simulink model "UNIFIER_3DOFsim"  (R2023b)
settings: Solver=VariableStepAuto  StartTime=0  StopTime=t_sim  RelTol=1e-3
InitFcn:
  | UNIFIER_3DOFsim_init
values from neighbouring files (symbols this model uses):
  b = 20.11467    [UNIFIER_LOAD.m]    (also in UNIFIER_LOAD.mat; UNIFIER_LOAD_ROM.m; UNIFIER_LOAD_ROM.mat)
  c = 1.43676    [UNIFIER_LOAD.m]    (also in UNIFIER_LOAD.mat; UNIFIER_LOAD_ROM.m; UNIFIER_LOAD_ROM.mat)
  DEP_inc = -0.0872664625997    [UNIFIER_LOAD.mat]    (also in UNIFIER_ROMdyn.m = deg2rad(-5); UNIFIER_ROMdyn_script.m = deg2rad(-5); UNIFIER_ROMdyn_v2.m = deg2rad(-5); UNIFIER_ROMgen.m = 0.1)
  dp_DEP =     [UNIFIER_LOAD.mat]    (also in UNIFIER_LOAD_ROM.mat)
  dp_FUSE_FIN =     [UNIFIER_LOAD.mat]
  dp_HTU =     [UNIFIER_LOAD.mat]    (also in UNIFIER_LOAD_ROM.mat)
  dp_VTAIL =     [UNIFIER_LOAD.mat]
  dp_VTAIL_INDUCED =     [UNIFIER_LOAD.mat]
  dp_WING_root =     [UNIFIER_LOAD.mat]
  dp_WING_tip =     [UNIFIER_LOAD.mat]
  dumax = [2.09439510239 2.09439510239 2.09439510239 1.0471975512 2 4 2]    [UNIFIER_LOAD.mat]    (also in UNIFIER_LOAD_ROM.mat = [1.0471975512 1.0471975512 1.0471975512 0.174532925199 2 2 2)
  gr = 9.80665    [UNIFIER_LOAD.mat]    (also in UNIFIER_LOAD_ROM.mat)
  m = 7057    [UNIFIER_LOAD.m]    (also in UNIFIER_LOAD.mat; UNIFIER_LOAD_ROM.m; UNIFIER_LOAD_ROM.mat)
  n_prop = 12    [UNIFIER_LOAD.mat]    (also in UNIFIER_ROMdyn.m; UNIFIER_ROMdyn_script.m; UNIFIER_ROMdyn_v2.m)
  prop_d = 1.6    [UNIFIER_LOAD.mat]    (also in UNIFIER_ROMdyn.m; UNIFIER_ROMdyn_script.m; UNIFIER_ROMdyn_v2.m)
  ROMv1 = ROM    [UNIFIER_3DOFsim_init.m]    (also in UNIFIER_ROMgen_subset.m; UNIFIER_ROMgen_v2_subset.m; UNIFIER_ROMgen_v3_subset.m; UNIFIER_ROMgen_v4_subset.m)
  ROMv2 = ROM    [UNIFIER_3DOFsim_init.m]
  ROMv3 = ROM    [UNIFIER_3DOFsim_init.m]
  S = 29.98388    [UNIFIER_LOAD.m]    (also in UNIFIER_LOAD.mat; UNIFIER_LOAD_ROM.m; UNIFIER_LOAD_ROM.mat)
  U_trim = [ustar(3) ... (first row only)    [UNIFIER_3DOFsim_init.m]
  umax = inf    [UNIFIERLanding.m]    (also in UNIFIER_LOAD.mat = [0.436332312999 0.523598775598 0.523598775598 0.436332312999; UNIFIER_LOAD_ROM.mat = [0.436332312999 0.523598775598 0.349065850399 0.436332312999)
  umin = 0    [UNIFIERLanding.m]    (also in UNIFIER_LOAD.mat = [-0.436332312999 -0.523598775598 -0.523598775598 0 0 -1 -0.5; UNIFIER_LOAD_ROM.mat = [-0.436332312999 -0.523598775598 -0.0872664625997 0 0 -1 0])
  Va = sqrt(u^2+w^2)    [ROMcomp.m]    (also in UNIFIERLanding.m = sqrt(x(:,3).^2+x(:,4).^2); UNIFIERLanding_Dynamics_Internal.m = sqrt(X(:,3).^2+X(:,4).^2); UNIFIERLanding_Main.m = sqrt(solution.X(:,3).^2+solution.X(:,4).^2); UNIFIERLanding_trajopt.m = sqrt(solution.X(:,3).^2+solution.X(:,4).^2))
  vtail_nodes = [dp_VTAIL.Xs_LE;     dp_VTAIL.Ys_LE;     dp_VTAIL.Zs_LE]    [UNIFIER_LOAD.m]    (also in UNIFIER_LOAD.mat = [-16.4894695282 -2.83441376686 -2.73765826225 -16.1370849609)
  wing_nodes = [fliplr(dp_WING_tip.LE_Xs),fliplr(dp_WING_root.LE_Xs),dp_WING_root.LE_Xs,dp_WING_tip.LE_Xs;     fliplr(-dp_WING_tip.LE_Ys),fliplr(-dp_WING_root.LE_Ys),dp_WING_root.LE_Ys,dp_WING_tip.LE_Ys;     fliplr(dp_WING_tip.LE_Zs),fliplr(dp_WING_root.LE_Zs),dp_WING_root.LE_Zs,dp_WING_tip.LE_Zs]    [UNIFIER_LOAD.m]    (also in UNIFIER_LOAD.mat = [-7.70795631409 -9.67500019073 -0.98178178072 -7.66801691055)
  x0 = xstar(1)    [UNIFIERLanding.m]    (also in UNIFIER_3DOFsim_init.m; UNIFIER_dynamics.m = x; UNIFIER_trim.m = [Va_target/100; UNIFIER_trim1.m = [Va_target)
  xstar = [0;        0;        -ze_target;        zstar(1)*100;        0;        zstar(2)*100;        0;        zstar(3);        0;        0;        0;        0]    [UNIFIER_trim.m]    (also in UNIFIER_trim0_res.mat = [0 0 -500 55.1327882403 0 -0.446351795968 0 1.36591182427e-0; UNIFIER_trim1.m = [0;        0;        -ze_target;        zstar(1);        0; ; UNIFIER_trim1_res.mat = [0 0 -1219 72.7310470326 0 1.14230710452 0 0.0157060522827 0; UNIFIER_trimHFM.m = [0;        0;        -runconfig.ze;        zstar(1)*100;    )
  xyz_cg = [-8.09,0,-0.2]    [UNIFIER_LOAD.m]    (also in UNIFIER_LOAD.mat = [-8.09 0 -0.2]; UNIFIER_LOAD_ROM.m; UNIFIER_LOAD_ROM.mat = [-8.09 0 -0.2])
  xyz_cg_12 = [-8.09 0 -0.2 -8.09 0 -0.2 -8.09 0 -0.2 -8.09 0 -0.2 ... (36 elements, 3x12)]    [UNIFIER_LOAD.mat]    (also in UNIFIER_LOAD_ROM.mat)
  xyz_DEP = [ -6.9629998	-6.9210000	-6.8660002	-6.8099999	-6.7540002	-6.6999998	-6.6999998	-6.7540002	-6.8099999	-6.8660002	-6.9210000	-6.9629998 ... (first row only)    [UNIFIER_LOAD.m]    (also in UNIFIER_LOAD.mat = [-6.9629998 -10.05 -0.90899998 -6.921 -8.4499998 -0.792 -6.8; UNIFIER_LOAD_ROM.m; UNIFIER_LOAD_ROM.mat = [-6.9629998 -10.05 -0.90899998 -6.921 -8.4499998 -0.792 -6.8)
  z0 = x(1,2)    [UNIFIERLanding.m]    (also in UNIFIER_3DOFsim_init.m = xstar(3); UNIFIER_trim.m = zstar; UNIFIER_trim1.m = zstar; UNIFIER_trimHFM.m = zstar)
undefined symbols (not defined in the file or in its folder): solution
libraries: simulink_extras x17, sharedutil x5, slpidlib x4, aerolibtransform2 x4, dspindex x2, matrix_library x1, shared6dof x1, aerolibatmos2 x1, simulink x1
(part 2 of 4)

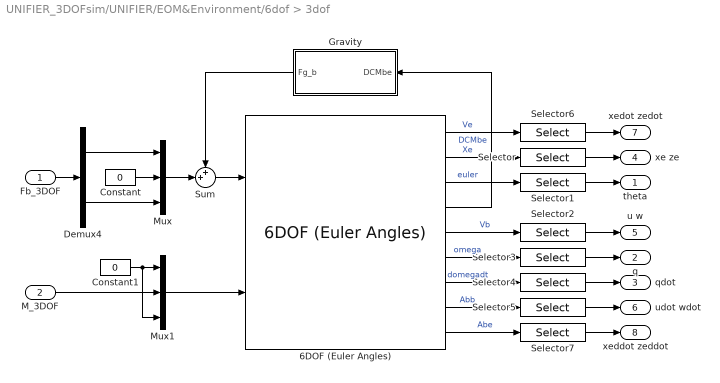
== system UNIFIER_3DOFsim/UNIFIER/EOM&Environment/6dof > 3dof ==
  Fb_3DOF : Inport
  M_3DOF : Inport  Port=2
  6DOF (Euler Angles) : shared6dof/6DOF (Euler Angles)  units=Metric (MKS)  mtype=Fixed  rep=Euler Angles  xme_0=Xe0  Vm_0=Vb0  eul_0=Euler0  pm_0=omegab0  mass_0=m  mass_e=0.5  mass_f=2.0  inertia=I  inertia_e=eye(3)  inertia_f=2*eye(3)  k_quat=1.0  vre_flag=on  abi_flag=on  aMode=0  xme_statename=''  Vm_statename=''  eul_statename=''  quat_statename=''  pm_statename=''  mass_statename=''
  Constant : Constant  Value=0
  Constant1 : Constant  Value=0
  Demux4 : Demux  Outputs=2
  Gravity : Subsystem
  Mux : Mux  Inputs=3
  Mux1 : Mux  Inputs=3
  Selector{,2,5..7} (5 alike) : Selector  InputPortWidth=3  IndexOptions=Index vector (dialog)  Indices=[1 3]  OutputSizes=1
  Selector1 : Selector  InputPortWidth=3  IndexOptions=Index vector (dialog)  Indices=[2]  OutputSizes=1
  Selector3 : Selector  InputPortWidth=3  IndexOptions=Index vector (dialog)  Indices=[2]  OutputSizes=1
  Selector4 : Selector  InputPortWidth=3  IndexOptions=Index vector (dialog)  Indices=[2]  OutputSizes=1
  Sum : Sum  Inputs=++|
  theta : Outport
  q : Outport  Port=2
  qdot : Outport  Port=3
  xe ze : Outport  Port=4
  u w : Outport  Port=5
  udot wdot : Outport  Port=6
  xedot zedot : Outport  Port=7
  xeddot zeddot : Outport  Port=8
  wires:
  Fb_3DOF/1 -> Demux4/1
  6DOF (Euler Angles)/1 -> Selector6/1  "Ve"
  Constant/1 -> Mux/2
  6DOF (Euler Angles)/9 -> Selector7/1  "Abe"
  M_3DOF/1 -> Mux1/2
  Sum/1 -> 6DOF (Euler Angles)/1
  Demux4/1 -> Mux/1
  Mux1/1 -> 6DOF (Euler Angles)/2
  Demux4/2 -> Mux/3
  Mux/1 -> Sum/2
  Gravity/1(Fg_b) -> Sum/1
  6DOF (Euler Angles)/2 -> Selector/1  "Xe"
  6DOF (Euler Angles)/4 -> Gravity/1(DCMbe)  "DCMbe"
  Constant1/1 -> Mux1/3, Mux1/1
  6DOF (Euler Angles)/3 -> Selector1/1  "euler"
  6DOF (Euler Angles)/5 -> Selector2/1  "Vb"
  6DOF (Euler Angles)/6 -> Selector3/1  "omega"
  6DOF (Euler Angles)/7 -> Selector4/1  "domegadt"
  6DOF (Euler Angles)/8 -> Selector5/1  "Abb"
  Selector/1 -> xe ze/1
  Selector1/1 -> theta/1
  Selector2/1 -> u w/1
  Selector3/1 -> q/1
  Selector4/1 -> qdot/1
  Selector5/1 -> udot wdot/1
  Selector6/1 -> xedot zedot/1
  Selector7/1 -> xeddot zeddot/1

== system UNIFIER_3DOFsim/UNIFIER/EOM&Environment/AlphaGammaVa ==
  uw : Inport
  theta : Inport  Port=2
  rho : Inport  Port=3
  Atan2 : Trigonometry  Operator=atan2
  Demux : Demux  Outputs=2
  Dot Product : DotProduct  OutDataTypeStr=Inherit: Inherit via internal rule
  Gain : Gain  Gain=1/1.225
  Product : Product
  Sqrt : Sqrt
  Sqrt1 : Sqrt
  Sum : Sum  Inputs=|+-
  alpha : Outport
  gamma : Outport  Port=2
  Va_tas : Outport  Port=3
  Va_eas : Outport  Port=4
  wires:
  uw/1 -> Dot Product/2, Dot Product/1, Demux/1
  Demux/2 -> Atan2/1
  Atan2/1 -> Sum/2, alpha/1
  theta/1 -> Sum/1
  Sum/1 -> gamma/1
  Demux/1 -> Atan2/2
  Dot Product/1 -> Sqrt/1
  Sqrt/1 -> Product/1, Va_tas/1
  Sqrt1/1 -> Product/2
  Product/1 -> Va_eas/1
  Gain/1 -> Sqrt1/1
  rho/1 -> Gain/1

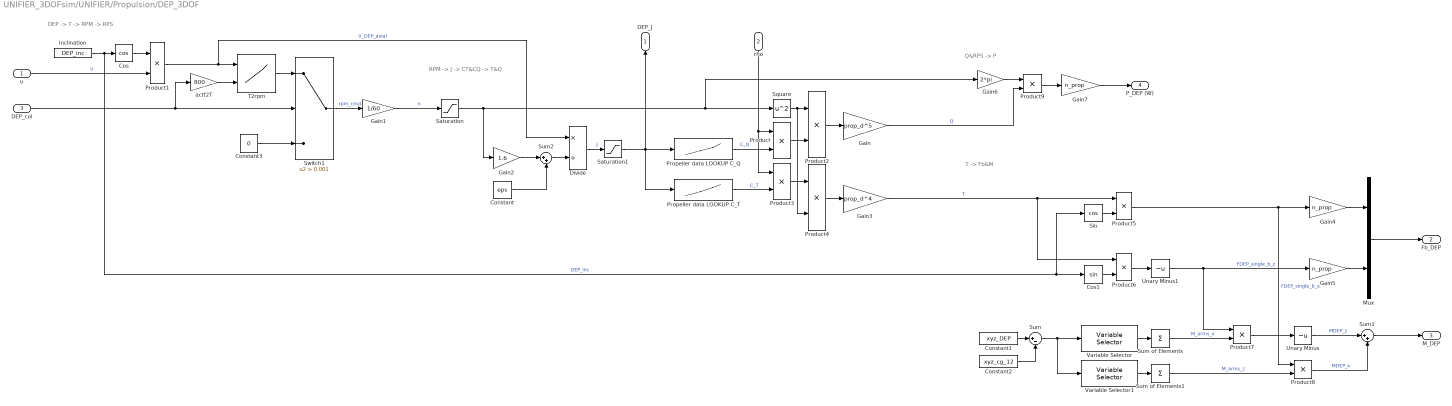
== system UNIFIER_3DOFsim/UNIFIER/Propulsion/DEP_3DOF ==
  note: Q&RPS -> P
  note: T -> Fb&M
  note: RPM -> J -> CT&CQ -> T&Q
  note: DEP -> T -> RPM -> RPS
  u : Inport
  rho : Inport  Port=2
  DEP_col : Inport  Port=3
  Constant : Constant  Value=eps
  Constant1 : Constant  Value=xyz_DEP
  Constant2 : Constant  Value=xyz_cg_12
  Constant3 : Constant  Value=0
  Cos : Trigonometry  Operator=cos
  Cos1 : Trigonometry
  Divide : Product  Inputs=*/
  Gain : Gain  Gain=prop_d^5
  Gain1 : Gain  Gain=1/60
  Gain2 : Gain  Gain=1.6
  Gain3 : Gain  Gain=prop_d^4
  Gain4 : Gain  Gain=n_prop
  Gain5 : Gain  Gain=n_prop
  Gain6 : Gain  Gain=2*pi
  Gain7 : Gain  Gain=n_prop
  Inclination : Constant  Value=DEP_inc
  Mux : Mux  Inputs=2
  Product{,1..9} (10 alike) : Product
  Propeller data LOOKUP C_Q : Lookup_n-D  NumberOfTableDimensions=1  BreakpointsForDimension1=dp_DEP.J  IndexSearchMethod=Linear search  BeginIndexSearchUsingPreviousIndexResult=on  Table=dp_DEP.C_Q  ExtrapMethod=Clip  UseLastTableValue=on  InternalRulePriority=Speed  RndMeth=Simplest
  Propeller data LOOKUP C_T : Lookup_n-D  NumberOfTableDimensions=1  BreakpointsForDimension1=dp_DEP.J  IndexSearchMethod=Linear search  BeginIndexSearchUsingPreviousIndexResult=on  Table=dp_DEP.C_T  ExtrapMethod=Clip  UseLastTableValue=on  InternalRulePriority=Speed  RndMeth=Simplest
  Saturation : Saturate  UpperLimit=inf  LowerLimit=0
  Saturation1 : Saturate  UpperLimit=2.5  LowerLimit=0.3
  Sin : Trigonometry  Operator=cos
  Square : Math  Operator=square
  Sum : Sum  Inputs=|+-
  Sum of Elements : Sum  Inputs=+
  Sum of Elements1 : Sum  Inputs=+
  Sum1 : Sum  Inputs=|++
  Sum2 : Sum  Inputs=|++
  Switch1 : Switch  Criteria=u2 > Threshold  Threshold=0.001  SaturateOnIntegerOverflow=off  InputSameDT=off
  T2rpm : Lookup_n-D  BreakpointsForDimension1=dp_DEP.rpm_lookup.V_vec  BreakpointsForDimension2=dp_DEP.rpm_lookup.T_vec  IndexSearchMethod=Linear search  BeginIndexSearchUsingPreviousIndexResult=on  Table=dp_DEP.rpm_lookup.rpm_gird  ExtrapMethod=Clip  InternalRulePriority=Speed  RndMeth=Simplest
      settings: InputPortMap=u0,u1
  Unary Minus : UnaryMinus
  Unary Minus1 : UnaryMinus
  Variable Selector : dspindex/Variable Selector  NumInputs=1  rowsOrCols=Rows  IdxMode=Fixed  Elements=[1]  ZerOneIdxMode=One-based  errmode=Clip Index  FillMode=on  FillValues=0
  Variable Selector1 : dspindex/Variable Selector  NumInputs=1  rowsOrCols=Rows  IdxMode=Fixed  Elements=[3]  ZerOneIdxMode=One-based  errmode=Clip Index  FillMode=on  FillValues=0
  actf2T : Gain  Gain=800
  DEP_J : Outport
  Fb_DEP : Outport  Port=2
  M_DEP : Outport  Port=3
  P_DEP (W) : Outport  Port=4
  wires:
  Cos/1 -> Product1/1
  Inclination/1 -> Cos1/1, Sin/1, Cos/1  "DEP_inc"
  u/1 -> Product1/2  "u"
  Constant2/1 -> Sum/2
  Constant1/1 -> Sum/1
  Constant3/1 -> Switch1/3
  T2rpm/1 -> Switch1/1
  actf2T/1 -> T2rpm/2
  Product1/1 -> Divide/1, T2rpm/1  "V_DEP_axial"
  DEP_col/1 -> actf2T/1, Switch1/2
  Switch1/1 -> Gain1/1  "rpm_cmd"
  Gain1/1 -> Saturation/1  "n"
  Product2/1 -> Gain/1
  Product4/1 -> Gain3/1
  Gain3/1 -> Product6/1, Product5/1  "T"
  Gain2/1 -> Sum2/1
  Constant/1 -> Sum2/2
  Gain/1 -> Product9/2  "Q"
  Saturation/1 -> Gain2/1, Square/1, Gain6/1
  Divide/1 -> Saturation1/1  "J"
  Saturation1/1 -> Propeller data LOOKUP C_Q/1, Propeller data LOOKUP C_T/1, DEP_J/1
  Product/1 -> Product2/2
  Propeller data LOOKUP C_T/1 -> Product3/2  "C_T"
  Propeller data LOOKUP C_Q/1 -> Product/2  "C_Q"
  Square/1 -> Product2/1, Product4/2
  Product3/1 -> Product4/1
  rho/1 -> Product/1, Product3/1
  Sum2/1 -> Divide/2
  Sum/1 -> Variable Selector1/1, Variable Selector/1
  Variable Selector/1 -> Sum of Elements/1
  Variable Selector1/1 -> Sum of Elements1/1
  Sum of Elements/1 -> Product7/2  "M_arms_x"
  Sum of Elements1/1 -> Product8/2  "M_arms_z"
  Sin/1 -> Product5/2
  Cos1/1 -> Product6/2
  Product5/1 -> Product8/1, Gain4/1  "FDEP_single_b_x"
  Product6/1 -> Unary Minus1/1
  Unary Minus1/1 -> Product7/1, Gain5/1  "FDEP_single_b_z"
  Gain4/1 -> Mux/1
  Gain5/1 -> Mux/2
  Mux/1 -> Fb_DEP/1
  Product7/1 -> Unary Minus/1
  Unary Minus/1 -> Sum1/1  "MDEP_z"
  Product8/1 -> Sum1/2  "MDEP_x"
  Sum1/1 -> M_DEP/1
  Gain6/1 -> Product9/1
  Product9/1 -> Gain7/1
  Gain7/1 -> P_DEP (W)/1

== system UNIFIER_3DOFsim/UNIFIER/Propulsion/HTU ==
  Va_eas : Inport
  HTU : Inport  Port=2
  1-D Lookup Table1 : Lookup_n-D  NumberOfTableDimensions=1  BreakpointsForDimension1=[-0.5,1.5]  IndexSearchMethod=Linear search  BeginIndexSearchUsingPreviousIndexResult=on  Table=[-5000, 15000]  ExtrapMethod=Clip  InternalRulePriority=Speed  RndMeth=Simplest
  Constant : Constant  Value=0
  Gain : Gain  Gain=1/0.92
  Gain1 : Gain  Gain=1000
  Mux : Mux  Inputs=2
  PropAndMotor : Subsystem
  Fb_HTU : Outport
  M_HTU : Outport  Port=2
  P_HTU (W) : Outport  Port=3
  wires:
  Gain/1 -> Gain1/1  "P(kW)"
  HTU/1 -> 1-D Lookup Table1/1
  1-D Lookup Table1/1 -> PropAndMotor/2(T_cmd (N))
  Va_eas/1 -> PropAndMotor/1(Vrw_mag_eas)
  PropAndMotor/1(P (kW)) -> Gain/1
  PropAndMotor/2(T (N)) -> Mux/1
  Mux/1 -> Fb_HTU/1
  Constant/1 -> M_HTU/1, Mux/2
  Gain1/1 -> P_HTU (W)/1

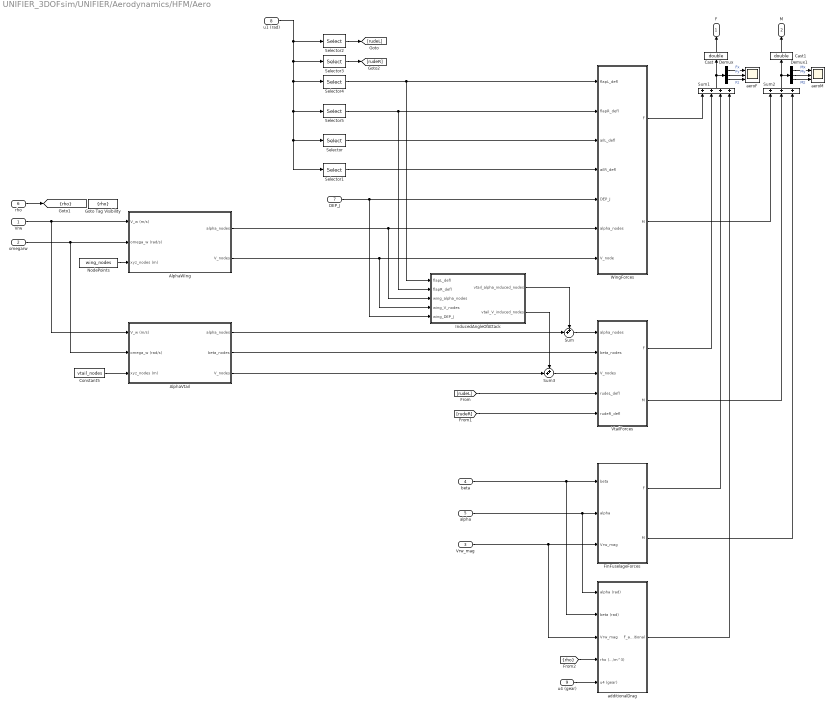
== system UNIFIER_3DOFsim/UNIFIER/Aerodynamics/HFM/Aero ==
  Vrw : Inport  OutDataTypeStr=single  Unit=m/s  PortDimensions=3  LockScale=on
  omegarw : Inport  Port=2  OutDataTypeStr=single  Unit=rad/s  PortDimensions=3  LockScale=on
  Vrw_mag : Inport  Port=3  OutDataTypeStr=single
  beta : Inport  Port=4  OutDataTypeStr=single
  alpha : Inport  Port=5  OutDataTypeStr=single
  rho : Inport  Port=6  OutDataTypeStr=single  Unit=kg/m^3  PortDimensions=1  LockScale=on
  DEP_J : Inport  Port=7  OutDataTypeStr=single  PortDimensions=12  LockScale=on
  u1 (rad) : Inport  Port=8
  u4 (gear) : Inport  Port=9
  AlphaVtail : Subsystem  TreatAsAtomicUnit=on
  AlphaWIng : Subsystem  TreatAsAtomicUnit=on
  Cast : DataTypeConversion  OutDataTypeStr=double  SaturateOnIntegerOverflow=off  RndMeth=Floor
  Cast1 : DataTypeConversion  OutDataTypeStr=double  SaturateOnIntegerOverflow=off  RndMeth=Floor
  Constant5 : Constant  Value=vtail_nodes
  Demux : Demux  Outputs=3
  Demux1 : Demux  Outputs=3
  FinFuselageForces : Subsystem
  Goto Tag Visibility : GotoTagVisibility  GotoTag=rho
  InducedAngleOfAttack : Subsystem
  NodePoints : Constant  Value=wing_nodes
  Selector : Selector  InputPortWidth=6  IndexOptions=Index vector (dialog)  Indices=1  OutputSizes=1
  Selector1 : Selector  InputPortWidth=6  IndexOptions=Index vector (dialog)  Indices=2  OutputSizes=1
  Selector2 : Selector  InputPortWidth=6  IndexOptions=Index vector (dialog)  Indices=3  OutputSizes=1
  Selector3 : Selector  InputPortWidth=6  IndexOptions=Index vector (dialog)  Indices=4  OutputSizes=1
  Selector4 : Selector  InputPortWidth=6  IndexOptions=Index vector (dialog)  Indices=5  OutputSizes=1
  Selector5 : Selector  InputPortWidth=6  IndexOptions=Index vector (dialog)  Indices=6  OutputSizes=1
  Sum : Sum  Inputs=++|
  Sum1 : Sum  Inputs=++++
  Sum2 : Sum  Inputs=+++
  Sum3 : Sum  Inputs=++|
  VtailForces : Subsystem
  WingForces : Subsystem
  additionalDrag : Subsystem
  aeroF : Scope  NumInputPorts=3
  aeroM : Scope  NumInputPorts=3
  F : Outport  Unit=N  PortDimensions=3  LockScale=on
  M : Outport  Port=2  Unit=N*m  PortDimensions=3  LockScale=on
  tag scope: rho=scoped
  wires:
  u1 (rad)/1 -> Selector2/1, Selector3/1, Selector4/1, Selector5/1, Selector/1, Selector1/1
  u4 (gear)/1 -> additionalDrag/5(u4 (gear))
  additionalDrag/1(F_additional) -> Sum1/4
  [rho] -> additionalDrag/4(rho (kg/m^3))
  alpha/1 -> FinFuselageForces/2(alpha), additionalDrag/1(alpha (rad))
  AlphaWIng/1(alpha_nodes) -> InducedAngleOfAttack/3(wing_alpha_nodes), WingForces/6(alpha_nodes)
  Demux1/3 -> aeroM/3  "Mz"
  Demux1/1 -> aeroM/1  "Mx"
  Demux1/2 -> aeroM/2  "My"
  Sum2/1 -> Demux1/1, Cast1/1
  Demux/3 -> aeroF/3  "Fz"
  Demux/2 -> aeroF/2  "Fy"
  Demux/1 -> aeroF/1  "Fx"
  Selector3/1 -> [rudeR]
  Selector2/1 -> [rudeL]
  Selector5/1 -> InducedAngleOfAttack/2(flapR_defl), WingForces/2(flapR_defl)
  Selector4/1 -> InducedAngleOfAttack/1(flapL_defl), WingForces/1(flapL_defl)
  Selector1/1 -> WingForces/4(ailR_defl)
  Selector/1 -> WingForces/3(ailL_defl)
  FinFuselageForces/2(M) -> Sum2/3
  FinFuselageForces/1(F) -> Sum1/3
  beta/1 -> FinFuselageForces/1(beta), additionalDrag/2(beta (rad))
  Vrw_mag/1 -> FinFuselageForces/3(Vrw_mag), additionalDrag/3(Vrw_mag)
  Cast1/1 -> M/1
  Cast/1 -> F/1
  AlphaVtail/1(alpha_nodes) -> Sum/2
  Sum3/1 -> VtailForces/3(V_nodes)
  InducedAngleOfAttack/2(vtail_V_induced_nodes) -> Sum3/1
  InducedAngleOfAttack/1(vtail_alpha_induced_nodes) -> Sum/1
  AlphaVtail/3(V_nodes) -> Sum3/2
  Sum1/1 -> Cast/1, Demux/1
  VtailForces/2(M) -> Sum2/2
  WingForces/2(M) -> Sum2/1
  VtailForces/1(F) -> Sum1/2
  WingForces/1(F) -> Sum1/1
  [rudeR] -> VtailForces/5(rudeR_defl)
  [rudeL] -> VtailForces/4(rudeL_defl)
  AlphaVtail/2(beta_nodes) -> VtailForces/2(beta_nodes)
  rho/1 -> [rho]
  Sum/1 -> VtailForces/1(alpha_nodes)
  DEP_J/1 -> InducedAngleOfAttack/5(wing_DEP_J), WingForces/5(DEP_J)
  AlphaWIng/2(V_nodes) -> InducedAngleOfAttack/4(wing_V_nodes), WingForces/7(V_node)
  omegarw/1 -> AlphaWIng/2(omega_w (rad/s)), AlphaVtail/2(omega_w (rad/s))
  Vrw/1 -> AlphaWIng/1(V_w (m/s)), AlphaVtail/1(V_w (m/s))
  Constant5/1 -> AlphaVtail/3(xyz_nodes (m))
  NodePoints/1 -> AlphaWIng/3(xyz_nodes (m))

== system UNIFIER_3DOFsim/UNIFIER/Aerodynamics/HFM/FillControls ==
  U_3dof : Inport
  Constant : Constant  Value=0
  Demux : Demux
  Mux : Mux  Inputs=7
  U_6dof : Outport
  wires:
  Constant/1 -> Mux/1, Mux/2, Mux/6  "ail, rud, DEP_slp"
  Mux/1 -> U_6dof/1
  U_3dof/1 -> Demux/1
  Demux/1 -> Mux/3  "elev"
  Demux/2 -> Mux/4  "flap"
  Demux/3 -> Mux/5  "DEP_col"
  Demux/4 -> Mux/7  "HTU"

== system UNIFIER_3DOFsim/UNIFIER/Aerodynamics/HFM/FillStates ==
  X_3dof : Inport
  Bus Selector : BusSelector  OutputSignals=q,theta,w,u,ze,xe
  Constant : Constant  Value=0
  Mux : Mux  Inputs=12
  X_6dof : Outport
  wires:
  X_3dof/1 -> Bus Selector/1
  Bus Selector/6 -> Mux/1  "<xe>"
  Mux/1 -> X_6dof/1
  Bus Selector/5 -> Mux/3  "<ze>"
  Bus Selector/4 -> Mux/4  "<u>"
  Bus Selector/3 -> Mux/6  "<w>"
  Bus Selector/2 -> Mux/8  "<theta>"
  Bus Selector/1 -> Mux/11  "<q>"
  Constant/1 -> Mux/12, Mux/10, Mux/9, Mux/5, Mux/2, Mux/7

== system UNIFIER_3DOFsim/UNIFIER/Aerodynamics/HFM/Ganging ==
  U_ganged : Inport
  Constant : Constant  Value=0
  Demux : Demux  Outputs=7
  For Each Subsystem : Subsystem  TreatAsAtomicUnit=on
  Mux : Mux  Inputs=2
  Mux1 : Mux  Inputs=2
  Mux2 : Mux  Inputs=2
  Mux3 : Mux
  Mux4 : Mux  Inputs=3
  Unary Minus : UnaryMinus
  V-tail mixing : Subsystem
  zeta : Constant  Value=[-1, -0.8, -0.4, -0.2, -0.1, 0, 0, 0.1, 0.2, 0.4, 0.8, 1]
  U_all : Outport
  wires:
  U_ganged/1 -> Demux/1
  Mux3/1 -> U_all/1
  Demux/1 -> Mux/1, Unary Minus/1  "ail"
  Unary Minus/1 -> Mux/2
  V-tail mixing/1(rudL) -> Mux1/1
  V-tail mixing/2(rudR) -> Mux1/2
  Demux/4 -> Mux2/2, Mux2/1  "flap"
  Demux/7 -> Mux3/3  "u3"
  Mux/1 -> Mux4/1  "ail"
  Mux1/1 -> Mux4/2  "rud"
  Mux2/1 -> Mux4/3  "flap"
  Demux/5 -> For Each Subsystem/2(DEP_col)  "DEP_col"
  Demux/6 -> For Each Subsystem/3(DEP_slope)  "DEP_slp"
  For Each Subsystem/1(Out1) -> Mux3/2  "u2"
  Mux4/1 -> Mux3/1  "u1"
  Constant/1 -> Mux3/4  "u4"
  zeta/1 -> For Each Subsystem/1(zeta)
  Demux/2 -> V-tail mixing/1(rud)  "rud"
  Demux/3 -> V-tail mixing/2(elev)  "elev"

== system UNIFIER_3DOFsim/UNIFIER/Aerodynamics/HFM/Subsystem ==
  In1 : Inport
  Mux : Mux  Inputs=12
  Out1 : Outport
  wires:
  Mux/1 -> Out1/1
  In1/1 -> Mux/3, Mux/4, Mux/5, Mux/6, Mux/7, Mux/8, Mux/9, Mux/10, Mux/11, Mux/12, Mux/2, Mux/1

== system UNIFIER_3DOFsim/UNIFIER/Aerodynamics/ROM/ROMv1 ==
  alpha : Inport
  elev : Inport  Port=2
  flap : Inport  Port=3
  J : Inport  Port=4
  n-D Lookup Table : Lookup_n-D  NumberOfTableDimensions=4  BreakpointsForDimension1=ROMv1.dFlap  BreakpointsForDimension2=ROMv1.alpha  BreakpointsForDimension3=ROMv1.J  BreakpointsForDimension4=ROMv1.dElev  Table=ROMv1.CL  InternalRulePriority=Speed  RndMeth=Simplest
      settings: InputPortMap=u0,u1,u2,u3
  n-D Lookup Table1 : Lookup_n-D  NumberOfTableDimensions=4  BreakpointsForDimension1=ROMv1.dFlap  BreakpointsForDimension2=ROMv1.alpha  BreakpointsForDimension3=ROMv1.J  BreakpointsForDimension4=ROMv1.dElev  Table=ROMv1.CD  InternalRulePriority=Speed  RndMeth=Simplest
      settings: InputPortMap=u0,u1,u2,u3
  n-D Lookup Table2 : Lookup_n-D  NumberOfTableDimensions=4  BreakpointsForDimension1=ROMv1.dFlap  BreakpointsForDimension2=ROMv1.alpha  BreakpointsForDimension3=ROMv1.J  BreakpointsForDimension4=ROMv1.dElev  Table=ROMv1.CM  InternalRulePriority=Speed  RndMeth=Simplest
      settings: InputPortMap=u0,u1,u2,u3
  CL : Outport
  CD : Outport  Port=2
  CM : Outport  Port=3
  wires:
  n-D Lookup Table/1 -> CL/1
  n-D Lookup Table1/1 -> CD/1
  n-D Lookup Table2/1 -> CM/1
  flap/1 -> n-D Lookup Table/1, n-D Lookup Table2/1, n-D Lookup Table1/1
  alpha/1 -> n-D Lookup Table/2, n-D Lookup Table2/2, n-D Lookup Table1/2
  J/1 -> n-D Lookup Table2/3, n-D Lookup Table/3, n-D Lookup Table1/3
  elev/1 -> n-D Lookup Table2/4, n-D Lookup Table1/4, n-D Lookup Table/4

== system UNIFIER_3DOFsim/UNIFIER/Aerodynamics/ROM/ROMv2 ==
  alpha : Inport
  elev : Inport  Port=2
  flap : Inport  Port=3
  n-D Lookup Table : Lookup_n-D  NumberOfTableDimensions=3  BreakpointsForDimension1=ROMv2.alpha  BreakpointsForDimension2=ROMv2.dElev  BreakpointsForDimension3=ROMv2.dFlap  Table=ROMv2.CL  InternalRulePriority=Speed  RndMeth=Simplest
      settings: InputPortMap=u0,u1,u2
  n-D Lookup Table1 : Lookup_n-D  NumberOfTableDimensions=3  BreakpointsForDimension1=ROMv2.alpha  BreakpointsForDimension2=ROMv2.dElev  BreakpointsForDimension3=ROMv2.dFlap  Table=ROMv2.CD  InternalRulePriority=Speed  RndMeth=Simplest
      settings: InputPortMap=u0,u1,u2
  n-D Lookup Table2 : Lookup_n-D  NumberOfTableDimensions=3  BreakpointsForDimension1=ROMv2.alpha  BreakpointsForDimension2=ROMv2.dElev  BreakpointsForDimension3=ROMv2.dFlap  Table=ROMv2.CM  InternalRulePriority=Speed  RndMeth=Simplest
      settings: InputPortMap=u0,u1,u2
  CL : Outport
  CD : Outport  Port=2
  CM : Outport  Port=3
  wires:
  alpha/1 -> n-D Lookup Table/1, n-D Lookup Table2/1, n-D Lookup Table1/1
  elev/1 -> n-D Lookup Table2/2, n-D Lookup Table1/2, n-D Lookup Table/2
  flap/1 -> n-D Lookup Table2/3, n-D Lookup Table1/3, n-D Lookup Table/3
  n-D Lookup Table/1 -> CL/1
  n-D Lookup Table1/1 -> CD/1
  n-D Lookup Table2/1 -> CM/1

== system UNIFIER_3DOFsim/UNIFIER/Aerodynamics/ROM/ROMv3 ==
  alpha : Inport
  elev : Inport  Port=2
  1-D Lookup Table : Lookup_n-D  NumberOfTableDimensions=1  BreakpointsForDimension1=ROMv3.alpha  Table=ROMv3.CL  InternalRulePriority=Speed  RndMeth=Simplest
  1-D Lookup Table1 : Lookup_n-D  NumberOfTableDimensions=1  BreakpointsForDimension1=ROMv3.alpha  Table=ROMv3.CD  InternalRulePriority=Speed  RndMeth=Simplest
  2-D Lookup Table : Lookup_n-D  LookupTableObject=''  BreakpointsForDimension1=ROMv3.alpha  BreakpointsForDimension2=ROMv3.dElev  BreakpointsForDimension1FirstPoint=10  BreakpointsForDimension2FirstPoint=10  BreakpointsForDimension1Spacing=12  BreakpointsForDimension2Spacing=12  IndexSearchMethod=Evenly spaced points  Table=ROMv3.CM  InterpMethod=Flat  DiagnosticForOutOfRangeInput=Error  InternalRulePriority=Speed  RndMeth=Simplest
      settings: InputPortMap=u0,u1
  CL : Outport
  CD : Outport  Port=2
  CM : Outport  Port=3
  wires:
  alpha/1 -> 1-D Lookup Table/1, 2-D Lookup Table/1, 1-D Lookup Table1/1
  elev/1 -> 2-D Lookup Table/2
  1-D Lookup Table/1 -> CL/1
  1-D Lookup Table1/1 -> CD/1
  2-D Lookup Table/1 -> CM/1

== system UNIFIER_3DOFsim/UNIFIER/Aerodynamics/ROM/calcDynamicPresure ==
  rho : Inport
  Va : Inport  Port=2
  Gain : Gain  Gain=0.5
  Product : Product
  Square : Math  Operator=square
  Q : Outport
  wires:
  Va/1 -> Square/1
  Square/1 -> Product/1
  rho/1 -> Gain/1
  Gain/1 -> Product/2
  Product/1 -> Q/1

== system UNIFIER_3DOFsim/UNIFIER/Aerodynamics/ROM/wind2body ==
  L : Inport
  D : Inport  Port=2
  alpha : Inport  Port=3
  Cos : Trigonometry  Operator=cos
  Product{,1..3} (4 alike) : Product
  Sin : Trigonometry
  Sum : Sum  Inputs=|+-
  Sum1 : Sum  Inputs=|++
  Unary Minus : UnaryMinus
  Unary Minus1 : UnaryMinus
  Fb_ae_x : Outport
  Fb_ae_z : Outport  Port=2
  wires:
  alpha/1 -> Sin/1, Cos/1
  Unary Minus/1 -> Fb_ae_x/1
  Unary Minus1/1 -> Fb_ae_z/1
  Cos/1 -> Product3/1, Product/1
  D/1 -> Product/2, Product2/2
  Sin/1 -> Product1/1, Product2/1
  L/1 -> Product3/2, Product1/2
  Product/1 -> Sum/1  "Dcos(alpha)"
  Product1/1 -> Sum/2  "Lsin(alpha)"
  Sum/1 -> Unary Minus/1
  Product2/1 -> Sum1/1  "Dsin(alpha)"
  Product3/1 -> Sum1/2  "Lcos(alpha)"
  Sum1/1 -> Unary Minus1/1

== system UNIFIER_3DOFsim/UNIFIER/EOM&Environment/6dof > 3dof/Gravity ==
  DCMbe : Inport
  Constant1 : Constant  Value=m*gr
  Constant3 : Constant  Value=0
  Product3 : Product  Multiplication=Matrix(*)
  Vector Concatenate1 : Concatenate  NumInputs=3
  Fg_b : Outport
  wires:
  DCMbe/1 -> Product3/1
  Constant1/1 -> Vector Concatenate1/3
  Constant3/1 -> Vector Concatenate1/2, Vector Concatenate1/1
  Vector Concatenate1/1 -> Product3/2
  Product3/1 -> Fg_b/1  "F"

== system UNIFIER_3DOFsim/UNIFIER/Propulsion/HTU/PropAndMotor ==
  Vrw_mag_eas : Inport
  T_cmd (N) : Inport  Port=2
  1-D Lookup Table : Lookup_n-D  NumberOfTableDimensions=1  BreakpointsForDimension1=dp_HTU.limits.V_low_lim  IndexSearchMethod=Linear search  BeginIndexSearchUsingPreviousIndexResult=on  Table=dp_HTU.limits.T_low_lim  InternalRulePriority=Speed  RndMeth=Simplest
  1-D Lookup Table1 : Lookup_n-D  NumberOfTableDimensions=1  BreakpointsForDimension1=dp_HTU.limits.V_up_lim  IndexSearchMethod=Linear search  BeginIndexSearchUsingPreviousIndexResult=on  Table=dp_HTU.limits.T_up_lim  InternalRulePriority=Speed  RndMeth=Simplest
  P lookup : Lookup_n-D  BreakpointsForDimension1=dp_HTU.V_vec  BreakpointsForDimension2=dp_HTU.T_vec  IndexSearchMethod=Linear search  BeginIndexSearchUsingPreviousIndexResult=on  Table=dp_HTU.P_grid  InternalRulePriority=Speed  RndMeth=Simplest
      settings: InputPortMap=u0,u1
  Saturation Dynamic : simulink/Discontinuities/Saturation Dynamic  OutMin=[]  OutMax=[]  OutDataTypeStr=Inherit: Same as second input  OutDataType=fixdt(1, 16)  OutScaling=2^-10  DoSatur=off
  P (kW) : Outport
  T (N) : Outport  Port=2
  wires:
  Saturation Dynamic/1 -> P lookup/2, T (N)/1
  T_cmd (N)/1 -> Saturation Dynamic/2
  1-D Lookup Table/1 -> Saturation Dynamic/3
  1-D Lookup Table1/1 -> Saturation Dynamic/1
  P lookup/1 -> P (kW)/1
  Vrw_mag_eas/1 -> P lookup/1, 1-D Lookup Table1/1, 1-D Lookup Table/1

== system UNIFIER_3DOFsim/UNIFIER/Aerodynamics/HFM/Aero/AlphaVtail ==
  V_w (m/s) : Inport
  omega_w (rad/s) : Inport  Port=2
  xyz_nodes (m) : Inport  Port=3  Partition=on  PartitionDimension=2  PartitionWidth=1  PartitionOffset=0
  3x3 Cross Product : sharedutil/3x3 Cross Product  aMode=aMode
  Asin : Trigonometry  Operator=asin
  Atan : Trigonometry  Operator=atan
  Cast : DataTypeConversion  OutDataTypeStr=single  SaturateOnIntegerOverflow=off  RndMeth=Floor
  Constant : Constant  Value=xyz_cg
  Constant1 : Constant  Value=eps  OutDataTypeStr=single
  Demux : Demux  Outputs=3
  Divide : Product  Inputs=*/
  Divide1 : Product  Inputs=*/
  For Each : ForEach  DisableCoverage=on  SpecifiedNumIters=16
  Mux : Mux  Inputs=3
  Sum : Sum  Inputs=+-
  Sum1 : Sum  Inputs=++|
  Sum2 : Sum  Inputs=|++
  Sum3 : Sum  Inputs=|++
  V_inf : Fcn  Expr=sqrt(u(1)^2+u(2)^2+u(3)^2)
  alpha_nodes : Outport  ConcatenationDimension=2
  beta_nodes : Outport  Port=2  ConcatenationDimension=2
  V_nodes : Outport  Port=3  ConcatenationDimension=2
  wires:
  Cast/1 -> Sum/1
  Sum3/1 -> Divide1/2, V_nodes/1
  V_inf/1 -> Sum3/1
  Asin/1 -> beta_nodes/1  "beta"
  Mux/1 -> V_inf/1
  Demux/2 -> Divide1/1, Mux/2
  Divide1/1 -> Asin/1
  Constant1/1 -> Sum2/2, Sum3/2
  Sum2/1 -> Divide/2
  Atan/1 -> alpha_nodes/1
  Divide/1 -> Atan/1
  Demux/3 -> Divide/1, Mux/3  "w"
  Demux/1 -> Mux/1, Sum2/1  "u"
  Sum1/1 -> Demux/1
  V_w (m/s)/1 -> Sum1/2
  omega_w (rad/s)/1 -> 3x3 Cross Product/2
  xyz_nodes (m)/1 -> Sum/2
  Constant/1 -> Cast/1
  Sum/1 -> 3x3 Cross Product/1
  3x3 Cross Product/1 -> Sum1/1

== system UNIFIER_3DOFsim/UNIFIER/Aerodynamics/HFM/Aero/AlphaWIng ==
  V_w (m/s) : Inport
  omega_w (rad/s) : Inport  Port=2
  xyz_nodes (m) : Inport  Port=3  Partition=on  PartitionDimension=2  PartitionWidth=1  PartitionOffset=0
  Cast : DataTypeConversion  OutDataTypeStr=single  SaturateOnIntegerOverflow=off  RndMeth=Floor
  ComputeAlphaBetaV : Subsystem
  Constant : Constant  Value=xyz_cg
  Cross Product : matrix_library/Cross Product
  For Each : ForEach  DisableCoverage=on  SpecifiedNumIters=14
  Sum : Sum  Inputs=+-
  Sum1 : Sum  Inputs=++|
  Terminator : Terminator
  alpha_nodes : Outport  ConcatenationDimension=2
  V_nodes : Outport  Port=2  ConcatenationDimension=2
  wires:
  ComputeAlphaBetaV/1(alpha_nodes) -> alpha_nodes/1
  ComputeAlphaBetaV/2(beta_nodes) -> Terminator/1
  ComputeAlphaBetaV/3(V_nodes) -> V_nodes/1
  Sum1/1 -> ComputeAlphaBetaV/1(V_w_local)
  Cast/1 -> Sum/1
  V_w (m/s)/1 -> Sum1/2
  omega_w (rad/s)/1 -> Cross Product/2
  xyz_nodes (m)/1 -> Sum/2
  Constant/1 -> Cast/1
  Sum/1 -> Cross Product/1
  Cross Product/1 -> Sum1/1

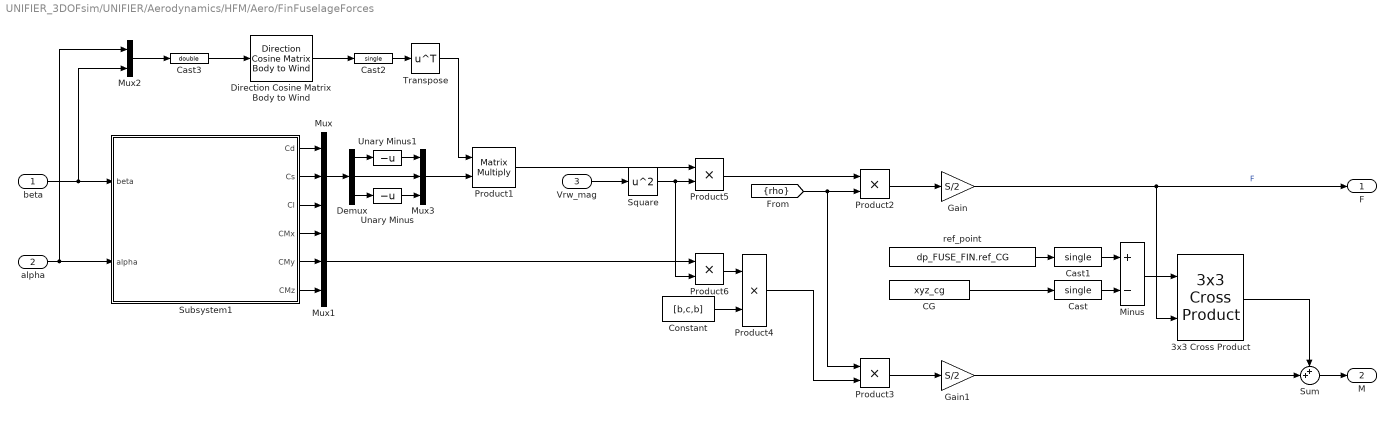
== system UNIFIER_3DOFsim/UNIFIER/Aerodynamics/HFM/Aero/FinFuselageForces ==
  beta : Inport
  alpha : Inport  Port=2
  Vrw_mag : Inport  Port=3  OutDataTypeStr=single
  3x3 Cross Product : sharedutil/3x3 Cross Product  aMode=aMode
  CG : Constant  Value=xyz_cg
  Cast : DataTypeConversion  OutDataTypeStr=single  SaturateOnIntegerOverflow=off  RndMeth=Floor
  Cast1 : DataTypeConversion  OutDataTypeStr=single  SaturateOnIntegerOverflow=off  RndMeth=Floor
  Cast2 : DataTypeConversion  OutDataTypeStr=single  SaturateOnIntegerOverflow=off  RndMeth=Floor
  Cast3 : DataTypeConversion  OutDataTypeStr=double  SaturateOnIntegerOverflow=off  RndMeth=Floor
  Constant : Constant  Value=[b,c,b]
  Demux : Demux  Outputs=3
  Direction Cosine Matrix Body to Wind : aerolibtransform2/Direction Cosine Matrix Body to Wind
  Gain : Gain  Gain=S/2
  Gain1 : Gain  Gain=S/2
  Minus : Sum  Inputs=+-
  Mux : Mux  Inputs=3
  Mux1 : Mux  Inputs=3
  Mux2 : Mux  Inputs=2
  Mux3 : Mux  Inputs=3
  Product1 : Product  Multiplication=Matrix(*)
  Product{2..6} (5 alike) : Product
  Square : Math  Operator=square
  Subsystem1 : Subsystem
  Sum : Sum  Inputs=++|
  Transpose : Math  Operator=transpose
  Unary Minus : UnaryMinus
  Unary Minus1 : UnaryMinus
  ref_point : Constant  Value=dp_FUSE_FIN.ref_CG
  F : Outport
  M : Outport  Port=2
  wires:
  Product2/1 -> Gain/1
  Product4/1 -> Product3/2
  Gain1/1 -> Sum/2
  [rho] -> Product2/2, Product3/1
  Constant/1 -> Product4/2
  Gain/1 -> F/1, 3x3 Cross Product/2  "F"
  Product3/1 -> Gain1/1
  Subsystem1/1(Cd) -> Mux/1
  Subsystem1/2(Cs) -> Mux/2
  Subsystem1/3(Cl) -> Mux/3
  Subsystem1/4(CMx) -> Mux1/1
  Subsystem1/5(CMy) -> Mux1/2
  Subsystem1/6(CMz) -> Mux1/3
  3x3 Cross Product/1 -> Sum/1
  ref_point/1 -> Cast1/1
  Cast/1 -> Minus/2
  Minus/1 -> 3x3 Cross Product/1
  CG/1 -> Cast/1
  Cast1/1 -> Minus/1
  beta/1 -> Mux2/2, Subsystem1/1(beta)
  alpha/1 -> Mux2/1, Subsystem1/2(alpha)
  Sum/1 -> M/1
  Mux2/1 -> Cast3/1
  Transpose/1 -> Product1/1
  Direction Cosine Matrix Body to Wind/1 -> Cast2/1
  Cast3/1 -> Direction Cosine Matrix Body to Wind/1
  Cast2/1 -> Transpose/1
  Demux/1 -> Unary Minus1/1
  Demux/2 -> Mux3/2
  Demux/3 -> Unary Minus/1
  Mux3/1 -> Product1/2
  Unary Minus/1 -> Mux3/3
  Unary Minus1/1 -> Mux3/1
  Square/1 -> Product6/2, Product5/2
  Product1/1 -> Product5/1
  Vrw_mag/1 -> Square/1
  Product5/1 -> Product2/1
  Mux1/1 -> Product6/1
  Product6/1 -> Product4/1
  Mux/1 -> Demux/1

== system UNIFIER_3DOFsim/UNIFIER/Aerodynamics/HFM/Aero/InducedAngleOfAttack ==
  flapL_defl : Inport
  flapR_defl : Inport  Port=2
  wing_alpha_nodes : Inport  Port=3  PortDimensions=14
  wing_V_nodes : Inport  Port=4  PortDimensions=14
  wing_DEP_J : Inport  Port=5  PortDimensions=12
  1-D Lookup Table : Lookup_n-D  NumberOfTableDimensions=1  BreakpointsForDimension1=wing_nodes(2,5:10)  BeginIndexSearchUsingPreviousIndexResult=on  TableSource=Input port  Table=tanh([-5:5])  ExtrapMethod=Clip  InternalRulePriority=Speed  RndMeth=Simplest
      settings: InputPortMap=u0,p221
  1-D Lookup Table1 : Lookup_n-D  NumberOfTableDimensions=1  BreakpointsForDimension1=wing_nodes(2,5:10)  BeginIndexSearchUsingPreviousIndexResult=on  TableSource=Input port  Table=tanh([-5:5])  ExtrapMethod=Clip  InternalRulePriority=Speed  RndMeth=Simplest
      settings: InputPortMap=u0,p221
  1-D Lookup Table2 : Lookup_n-D  NumberOfTableDimensions=1  BreakpointsForDimension1=wing_nodes(2,5:10)  BeginIndexSearchUsingPreviousIndexResult=on  TableSource=Input port  Table=tanh([-5:5])  ExtrapMethod=Clip  InternalRulePriority=Speed  RndMeth=Simplest
      settings: InputPortMap=u0,p221
  Constant : Constant  Value=ones(1,8)
  Constant1 : Constant  Value=ones(1,8)
  Constant7 : Constant  Value=vtail_nodes(2,:)
  Mux : Mux  Inputs=2
  Product : Product
  Product1 : Product
  Selector : Selector  InputPortWidth=14  IndexOptions=Index vector (dialog)  Indices=[5:10]  OutputSizes=1
  Selector1 : Selector  InputPortWidth=14  IndexOptions=Index vector (dialog)  Indices=[5:10]  OutputSizes=1
  Selector2 : Selector  InputPortWidth=12  IndexOptions=Index vector (dialog)  Indices=[4:9]  OutputSizes=1
  V_induced : Interpolation_n-D  NumberOfTableDimensions=5  Table=dp_VTAIL_INDUCED.V_induced  NumSelectionDims=1  InternalRulePriority=Speed  TableDataTypeStr=Inherit: Inherit from 'Table data'
      settings: InputPortMap=u0,u1,u2,u3,u4,u5,u6,u7,u8
  alpha_induced : Interpolation_n-D  NumberOfTableDimensions=5  Table=dp_VTAIL_INDUCED.alpha_induced  NumSelectionDims=1  InternalRulePriority=Speed  TableDataTypeStr=Inherit: Inherit from 'Table data'
      settings: InputPortMap=u0,u1,u2,u3,u4,u5,u6,u7,u8
  preLook : Subsystem
  vtail_alpha_induced_nodes : Outport  PortDimensions=16
  vtail_V_induced_nodes : Outport  Port=2  PortDimensions=16
  wires:
  Selector2/1 -> 1-D Lookup Table2/2
  Selector1/1 -> 1-D Lookup Table1/2
  Selector/1 -> 1-D Lookup Table/2
  alpha_induced/1 -> vtail_alpha_induced_nodes/1
  V_induced/1 -> vtail_V_induced_nodes/1
  Mux/1 -> preLook/1(wing_flap_defl)
  Product1/1 -> Mux/2
  Product/1 -> Mux/1
  flapR_defl/1 -> Product1/2
  Constant1/1 -> Product1/1
  Constant/1 -> Product/1
  flapL_defl/1 -> Product/2
  wing_DEP_J/1 -> Selector2/1
  preLook/9(Out5) -> V_induced/9, alpha_induced/9
  preLook/8(Out7) -> V_induced/8, alpha_induced/8
  preLook/7(Out6) -> V_induced/7, alpha_induced/7
  preLook/6(Out4) -> V_induced/6, alpha_induced/6
  preLook/5(Out3) -> V_induced/5, alpha_induced/5
  preLook/4(Out9) -> V_induced/4, alpha_induced/4
  preLook/3(Out8) -> V_induced/3, alpha_induced/3
  preLook/2(Out2) -> V_induced/2, alpha_induced/2
  preLook/1(Out1) -> V_induced/1, alpha_induced/1
  wing_alpha_nodes/1 -> Selector/1
  wing_V_nodes/1 -> Selector1/1
  Constant7/1 -> 1-D Lookup Table1/1, 1-D Lookup Table2/1, 1-D Lookup Table/1
  1-D Lookup Table/1 -> preLook/2(wing_alphas)
  1-D Lookup Table2/1 -> preLook/4(wing_DEP_J)
  1-D Lookup Table1/1 -> preLook/3(wing_V_inf)

== system UNIFIER_3DOFsim/UNIFIER/Aerodynamics/HFM/Aero/VtailForces ==
  alpha_nodes : Inport  PortDimensions=16
  beta_nodes : Inport  Port=2  PortDimensions=16
  V_nodes : Inport  Port=3  PortDimensions=16
  rudeL_defl : Inport  Port=4
  rudeR_defl : Inport  Port=5
  Constant : Constant  Value=ones(1,8)
  Constant1 : Constant  Value=ones(1,8)
  Matrix Concatenate1 : Concatenate  NumInputs=3  Mode=Multidimensional array  ConcatenateDimension=2
  Matrix Concatenate2 : Concatenate  NumInputs=3  Mode=Multidimensional array  ConcatenateDimension=2
  Mux : Mux  Inputs=2
  Product : Product
  Product1 : Product
  Reshape : Reshape
  Reshape1 : Reshape
  Subsystem : Subsystem
  Transpose : Math  Operator=transpose
  Transpose1 : Math  Operator=transpose
  VtailForces : Subsystem
  F : Outport
  M : Outport  Port=2
  wires:
  Reshape1/1 -> F/1
  Reshape/1 -> M/1
  V_nodes/1 -> Subsystem/1(V_nodes)
  VtailForces/3(Cz) -> Matrix Concatenate1/3  "CFz"
  Subsystem/1(F) -> Reshape1/1
  Matrix Concatenate1/1 -> Transpose/1
  VtailForces/1(Cx) -> Matrix Concatenate1/1  "CFx"
  VtailForces/5(CMy) -> Matrix Concatenate2/2  "CMy"
  VtailForces/2(Cy) -> Matrix Concatenate1/2  "CFy"
  Transpose1/1 -> Subsystem/3(M_matrix)
  Transpose/1 -> Subsystem/2(F_matrix)
  Subsystem/2(M) -> Reshape/1
  Matrix Concatenate2/1 -> Transpose1/1
  VtailForces/6(CMz) -> Matrix Concatenate2/3  "CMz"
  VtailForces/4(CMx) -> Matrix Concatenate2/1  "CMx"
  rudeR_defl/1 -> Product1/2
  rudeL_defl/1 -> Product/2
  Constant/1 -> Product/1
  Constant1/1 -> Product1/1
  Mux/1 -> VtailForces/1(rude_defl_nodes)
  Product1/1 -> Mux/2
  Product/1 -> Mux/1
  beta_nodes/1 -> VtailForces/3(beta_nodes)
  alpha_nodes/1 -> VtailForces/2(alpha_nodes)

== system UNIFIER_3DOFsim/UNIFIER/Aerodynamics/HFM/Aero/WingForces ==
  flapL_defl : Inport
  flapR_defl : Inport  Port=2
  ailL_defl : Inport  Port=3
  ailR_defl : Inport  Port=4
  DEP_J : Inport  Port=5  PortDimensions=12
  alpha_nodes : Inport  Port=6  PortDimensions=14
  V_node : Inport  Port=7  PortDimensions=14
  Demux : Demux  Outputs=3
  Demux1 : Demux  Outputs=3
  Left : Subsystem
  Mux : Mux  Inputs=3
  Mux1 : Mux  Inputs=3
  Reshape : Reshape
  Reshape1 : Reshape
  Right : Subsystem
  Subsystem : Subsystem
  Sum : Sum  Inputs=|++
  Sum1 : Sum  Inputs=|++
  Unary Minus : UnaryMinus
  Unary Minus1 : UnaryMinus
  Unary Minus2 : UnaryMinus
  F : Outport
  M : Outport  Port=2
  wires:
  Reshape1/1 -> Sum1/2
  Reshape/1 -> Sum/2
  Subsystem/4(DEP_J_Right) -> Right/3(DEP_J)
  Subsystem/6(V_nodes_Right) -> Right/5(V_node)
  Subsystem/5(alpha_nodes_Right) -> Right/4(alpha)
  Right/2(M) -> Reshape1/1
  Right/1(F) -> Reshape/1
  Sum1/1 -> M/1
  Mux/1 -> Sum1/1
  Sum/1 -> F/1
  Mux1/1 -> Sum/1
  Demux/3 -> Mux1/3
  Demux/1 -> Mux1/1
  Unary Minus/1 -> Mux1/2
  Unary Minus2/1 -> Mux/3
  Unary Minus1/1 -> Mux/1
  Demux1/2 -> Mux/2
  Demux1/3 -> Unary Minus2/1
  Demux1/1 -> Unary Minus1/1
  Demux/2 -> Unary Minus/1
  Left/2(M) -> Demux1/1
  Left/1(F) -> Demux/1
  Subsystem/3(V_nodes_Left) -> Left/5(V_node)
  Subsystem/2(alpha_nodes_Left) -> Left/4(alpha)
  Subsystem/1(DEP_J_Left) -> Left/3(DEP_J)
  V_node/1 -> Subsystem/3(V_nodes)
  alpha_nodes/1 -> Subsystem/2(alpha_nodes)
  flapR_defl/1 -> Right/1(flap_defl)
  DEP_J/1 -> Subsystem/1(DEP_J)
  ailR_defl/1 -> Right/2(aile_defl)
  flapL_defl/1 -> Left/1(flap_defl)
  ailL_defl/1 -> Left/2(aile_defl)

== system UNIFIER_3DOFsim/UNIFIER/Aerodynamics/HFM/Aero/additionalDrag ==
  note: Wing mounted nacelles:
      | (Estimate using OpenVSP - Jenkinson Wing Mounted Nacelle)
      | =6*0.00043=0.00258
      | + cooling drag of 0.015
  note: Landing gear drag:
      | Loftin Jr, L. K. (1980). Subsonic aircraft: Evolution and the matching of size to performance (No. L-13367).
  alpha (rad) : Inport
  beta (rad) : Inport  Port=2
  Vrw_mag : Inport  Port=3
  rho (kg/m^3) : Inport  Port=4
  u4 (gear) : Inport  Port=5
  Cast : DataTypeConversion  OutDataTypeStr=single  SaturateOnIntegerOverflow=off  RndMeth=Floor
  Cast1 : DataTypeConversion  OutDataTypeStr=single  SaturateOnIntegerOverflow=off  RndMeth=Floor
  Cast2 : DataTypeConversion  OutDataTypeStr=double  SaturateOnIntegerOverflow=off  RndMeth=Floor
  Constant1 : Constant  Value=0  OutDataTypeStr=single
  Direction Cosine Matrix Body to Wind : aerolibtransform2/Direction Cosine Matrix Body to Wind
  Gain : Gain  Gain=S/2
  Math Function : Math  Operator=square
  Mux : Mux  Inputs=2
  Mux1 : Mux  Inputs=3
  Product : Product  OutDataTypeStr=single
  Product1 : Product  Multiplication=Matrix(*)
  Product2 : Product
  Product3 : Product
  Sum : Sum  Inputs=|++
  Transpose : Math  Operator=transpose
  Unary Minus : UnaryMinus
  extra_drag : Constant  Value=0.00258+0.015  OutDataTypeStr=single
  gear_drag : Constant  Value=0.015  OutDataTypeStr=single
  F_additional : Outport
  wires:
  Product3/1 -> Sum/2
  Sum/1 -> Product2/1
  gear_drag/1 -> Product3/1
  u4 (gear)/1 -> Product3/2
  Cast2/1 -> Direction Cosine Matrix Body to Wind/1
  Cast1/1 -> Transpose/1
  Cast/1 -> F_additional/1
  Product1/1 -> Cast/1
  Constant1/1 -> Mux1/3, Mux1/2
  Mux1/1 -> Product1/2
  Transpose/1 -> Product1/1
  Unary Minus/1 -> Mux1/1
  beta (rad)/1 -> Mux/2
  Mux/1 -> Cast2/1
  Direction Cosine Matrix Body to Wind/1 -> Cast1/1
  rho (kg/m^3)/1 -> Product2/2
  Vrw_mag/1 -> Math Function/1
  extra_drag/1 -> Sum/1
  Product2/1 -> Gain/1
  Gain/1 -> Product/1
  Product/1 -> Unary Minus/1
  Math Function/1 -> Product/2
  alpha (rad)/1 -> Mux/1

== system UNIFIER_3DOFsim/UNIFIER/Aerodynamics/HFM/Ganging/For Each Subsystem ==
  zeta : Inport  Partition=on  PartitionDimension=1  PartitionWidth=1  PartitionOffset=0
  DEP_col : Inport  Port=2
  DEP_slope : Inport  Port=3
  Add : Sum
  Display : Display
  For Each : ForEach  DisableCoverage=on
  K_slope : Gain  Gain=0.785
  Product : Product
  Tan : Trigonometry  Operator=tan
  Out1 : Outport  ConcatenationDimension=1
  wires:
  DEP_slope/1 -> K_slope/1
  K_slope/1 -> Tan/1
  Tan/1 -> Product/1
  zeta/1 -> Product/2
  Product/1 -> Add/1
  DEP_col/1 -> Add/2
  Add/1 -> Display/1, Out1/1

== system UNIFIER_3DOFsim/UNIFIER/Aerodynamics/HFM/Ganging/V-tail mixing ==
  rud : Inport
  elev : Inport  Port=2
  Sum : Sum  Inputs=|++
  Sum1 : Sum  Inputs=|++
  Unary Minus1 : UnaryMinus
  rudL : Outport
  rudR : Outport  Port=2
  wires:
  Sum/1 -> rudL/1
  Sum1/1 -> rudR/1
  rud/1 -> Sum1/2, Unary Minus1/1
  Unary Minus1/1 -> Sum/2
  elev/1 -> Sum1/1, Sum/1

== system UNIFIER_3DOFsim/UNIFIER/Aerodynamics/HFM/Aero/AlphaWIng/ComputeAlphaBetaV ==
  V_w_local : Inport
  Asin : Trigonometry  Operator=asin
  Atan : Trigonometry  Operator=atan
  Constant1 : Constant  Value=eps  OutDataTypeStr=single
  Demux : Demux  Outputs=3
  Divide : Product  Inputs=*/
  Divide1 : Product  Inputs=*/
  Dot Product : DotProduct  OutDataTypeStr=Inherit: Inherit via internal rule
  Square Root : Sqrt
  Sum2 : Sum  Inputs=|++
  alpha_nodes : Outport
  beta_nodes : Outport  Port=2
  V_nodes : Outport  Port=3
  wires:
  Atan/1 -> alpha_nodes/1
  Dot Product/1 -> Square Root/1
  Constant1/1 -> Sum2/2
  Asin/1 -> beta_nodes/1  "beta"
  Demux/3 -> Divide/1  "w"
  Divide/1 -> Atan/1
  Square Root/1 -> Divide1/2, V_nodes/1
  Sum2/1 -> Divide/2
  Demux/1 -> Sum2/1  "u"
  Divide1/1 -> Asin/1
  Demux/2 -> Divide1/1
  V_w_local/1 -> Demux/1, Dot Product/2, Dot Product/1

== system UNIFIER_3DOFsim/UNIFIER/Aerodynamics/HFM/Aero/FinFuselageForces/Subsystem1 ==
  beta : Inport
  alpha : Inport  Port=2
  Constant : Constant  Value=0  OutDataTypeStr=single
  Interpolation Using Prelookup : Interpolation_n-D  Table=dp_FUSE_FIN.CD  InternalRulePriority=Speed  TableDataTypeStr=single
  Interpolation Using Prelookup1 : Interpolation_n-D  Table=dp_FUSE_FIN.CS  InternalRulePriority=Speed
  Interpolation Using Prelookup3 : Interpolation_n-D  Table=dp_FUSE_FIN.CMx  InternalRulePriority=Speed
  Interpolation Using Prelookup4 : Interpolation_n-D  Table=dp_FUSE_FIN.CMy  InternalRulePriority=Speed
  Interpolation Using Prelookup5 : Interpolation_n-D  Table=dp_FUSE_FIN.CMz  InternalRulePriority=Speed
  Subsystem : Subsystem
  Cd : Outport
  Cs : Outport  Port=2
  Cl : Outport  Port=3
  CMx : Outport  Port=4
  CMy : Outport  Port=5
  CMz : Outport  Port=6
  wires:
  Subsystem/2(Out2) -> Interpolation Using Prelookup5/2, Interpolation Using Prelookup4/2, Interpolation Using Prelookup3/2, Interpolation Using Prelookup1/2, Interpolation Using Prelookup/2
  Subsystem/1(Out1) -> Interpolation Using Prelookup5/1, Interpolation Using Prelookup4/1, Interpolation Using Prelookup3/1, Interpolation Using Prelookup1/1, Interpolation Using Prelookup/1
  Subsystem/4(Out4) -> Interpolation Using Prelookup5/4, Interpolation Using Prelookup4/4, Interpolation Using Prelookup3/4, Interpolation Using Prelookup1/4, Interpolation Using Prelookup/4
  Interpolation Using Prelookup1/1 -> Cs/1
  alpha/1 -> Subsystem/2(alpha)
  Interpolation Using Prelookup4/1 -> CMy/1
  Subsystem/3(Out3) -> Interpolation Using Prelookup5/3, Interpolation Using Prelookup4/3, Interpolation Using Prelookup3/3, Interpolation Using Prelookup1/3, Interpolation Using Prelookup/3
  beta/1 -> Subsystem/1(beta)
  Interpolation Using Prelookup5/1 -> CMz/1
  Constant/1 -> Cl/1
  Interpolation Using Prelookup/1 -> Cd/1
  Interpolation Using Prelookup3/1 -> CMx/1

== system UNIFIER_3DOFsim/UNIFIER/Aerodynamics/HFM/Aero/InducedAngleOfAttack/preLook ==
  wing_flap_defl : Inport
  wing_alphas : Inport  Port=2
  wing_V_inf : Inport  Port=3
  wing_DEP_J : Inport  Port=4
  Constant8 : Constant  Value=0:15
  Prelookup : PreLookup  BreakpointsData=dp_VTAIL_INDUCED.flap_defl  IndexSearchMethod=Linear search  BeginIndexSearchUsingPreviousIndexResult=on  ExtrapMethod=Linear
  Prelookup1 : PreLookup  BreakpointsData=dp_VTAIL_INDUCED.V_infs  IndexSearchMethod=Linear search  BeginIndexSearchUsingPreviousIndexResult=on  ExtrapMethod=Linear
  Prelookup2 : PreLookup  BreakpointsData=dp_VTAIL_INDUCED.alphas  IndexSearchMethod=Linear search  BeginIndexSearchUsingPreviousIndexResult=on  ExtrapMethod=Linear
  Prelookup3 : PreLookup  BreakpointsData=dp_VTAIL_INDUCED.DEP_J  IndexSearchMethod=Linear search  BeginIndexSearchUsingPreviousIndexResult=on
  Out1 : Outport
  Out2 : Outport  Port=2
  Out8 : Outport  Port=3
  Out9 : Outport  Port=4
  Out3 : Outport  Port=5
  Out4 : Outport  Port=6
  Out6 : Outport  Port=7
  Out7 : Outport  Port=8
  Out5 : Outport  Port=9
  wires:
  Prelookup2/2 -> Out9/1
  Prelookup2/1 -> Out8/1
  Prelookup3/2 -> Out7/1
  Prelookup3/1 -> Out6/1
  wing_DEP_J/1 -> Prelookup3/1
  wing_alphas/1 -> Prelookup2/1
  wing_flap_defl/1 -> Prelookup/1
  Prelookup1/1 -> Out3/1
  wing_V_inf/1 -> Prelookup1/1
  Prelookup/2 -> Out2/1
  Prelookup1/2 -> Out4/1
  Constant8/1 -> Out5/1
  Prelookup/1 -> Out1/1

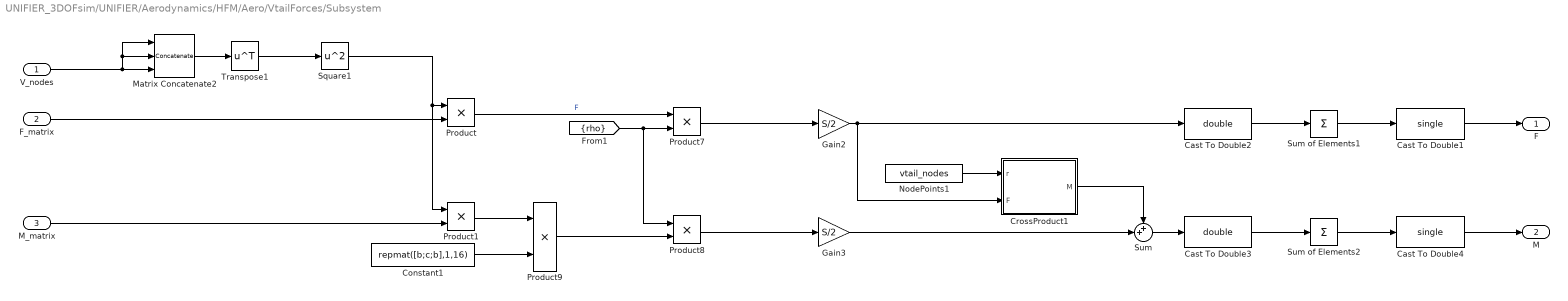
== system UNIFIER_3DOFsim/UNIFIER/Aerodynamics/HFM/Aero/VtailForces/Subsystem ==
  V_nodes : Inport
  F_matrix : Inport  Port=2
  M_matrix : Inport  Port=3
  Cast To Double1 : DataTypeConversion  OutDataTypeStr=single  SaturateOnIntegerOverflow=off  RndMeth=Floor
  Cast To Double2 : DataTypeConversion  OutDataTypeStr=double  SaturateOnIntegerOverflow=off  RndMeth=Floor
  Cast To Double3 : DataTypeConversion  OutDataTypeStr=double  SaturateOnIntegerOverflow=off  RndMeth=Floor
  Cast To Double4 : DataTypeConversion  OutDataTypeStr=single  SaturateOnIntegerOverflow=off  RndMeth=Floor
  Constant1 : Constant  Value=repmat([b;c;b],1,16)  VectorParams1D=off  OutDataTypeStr=single
  CrossProduct1 : Subsystem  TreatAsAtomicUnit=on
  Gain2 : Gain  Gain=S/2
  Gain3 : Gain  Gain=S/2
  Matrix Concatenate2 : Concatenate  NumInputs=3  Mode=Multidimensional array  ConcatenateDimension=2
  NodePoints1 : Constant  Value=vtail_nodes
  Product{,1,7..9} (5 alike) : Product
  Square1 : Math  Operator=square
  Sum : Sum  Inputs=++|
  Sum of Elements1 : Sum  Inputs=+  CollapseMode=Specified dimension  CollapseDim=2
  Sum of Elements2 : Sum  Inputs=+  CollapseMode=Specified dimension  CollapseDim=2
  Transpose1 : Math  Operator=transpose
  F : Outport
  M : Outport  Port=2
  wires:
  Cast To Double4/1 -> M/1
  Cast To Double3/1 -> Sum of Elements2/1
  Cast To Double1/1 -> F/1
  Cast To Double2/1 -> Sum of Elements1/1
  V_nodes/1 -> Matrix Concatenate2/3, Matrix Concatenate2/2, Matrix Concatenate2/1
  F_matrix/1 -> Product/2
  CrossProduct1/1(M) -> Sum/1
  Product1/1 -> Product9/1
  M_matrix/1 -> Product1/2
  Constant1/1 -> Product9/2
  Product8/1 -> Gain3/1
  [rho] -> Product7/2, Product8/1
  NodePoints1/1 -> CrossProduct1/1(r)
  Product9/1 -> Product8/2
  Gain3/1 -> Sum/2
  Matrix Concatenate2/1 -> Transpose1/1
  Square1/1 -> Product/1, Product1/1
  Product7/1 -> Gain2/1
  Product/1 -> Product7/1  "F"
  Transpose1/1 -> Square1/1
  Sum of Elements1/1 -> Cast To Double1/1
  Sum of Elements2/1 -> Cast To Double4/1
  Gain2/1 -> Cast To Double2/1, CrossProduct1/2(F)
  Sum/1 -> Cast To Double3/1
